simulink model "differentiator"  (R2020b)
settings: Solver=VariableStepAuto  StartTime=0.0  StopTime=0.2  MaxStep=1e-5  RelTol=1e-3  AbsTol=1e-3  EnableMultiTasking=on
libraries: fl_lib x9, nesl_utility x3
CloseFcn:
  | try,close(h1_ssc_opamp_differentiator),end
  | clear h1_ssc_opamp_differentiator
  | clear simlog_ssc_opamp_differentiator
Description:
  | Op-Amp Circuit - Differentiator
settings Model: Creator=The MathWorks, Inc.  LastModifiedBy=bolic
settings SolverCC: AutoScaleAbsTol=off
settings DataIOCC: LimitDataPoints=on  SaveFormat=Array  ReturnWorkspaceOutputs=off
settings OptimizationCC: LifeSpan=inf
settings DebuggingCC: SolverPrmCheckMsg=warning  AllowSymbolicDim=off  PregeneratedLibrarySubsystemCodeDiagnostic=none  SFUnexpectedBacktrackingDiag=warning  SFNoUnconditionalDefaultTransitionDiag=warning  SFExecutionAtInitializationDiag=none  ArithmeticOperatorsInVariantConditions=warning
settings HardwareCC: ProdBitPerPointer=32  ProdBitPerSizeT=32  ProdBitPerPtrDiffT=32  ProdLargestAtomicFloat=None  ProdIntDivRoundTo=Undefined  ProdEndianess=Unspecified  ProdWordSize=32  ProdHWDeviceType=32-bit Generic
settings ModelReferenceCC: PropagateSignalLabelsOutOfModel=off
settings SFSimCC: SimUseLocalCustomCode=off  CustomCodeUndefinedFunction=UseInterfaceOnly
settings RTWCC: RTWUseLocalCustomCode=off
settings CodeAppCC: StateflowObjectComments=on
settings GRTTargetCC: TargetLangStandard=C89/C90 (ANSI)
settings ConfigComp: CovMetricSettings=dw  CovSaveCumulativeToWorkspaceVar=on  CovSaveSingleToWorkspaceVar=on  CovExternalEMLEnable=off  CovSFcnEnable=off
settings SimscapeCC: SimscapeLogType=all  SimscapeLogSimulationStatistics=on  SimscapeLogName=simlog_ssc_opamp_differentiator  SimscapeLogDataHistory=10000

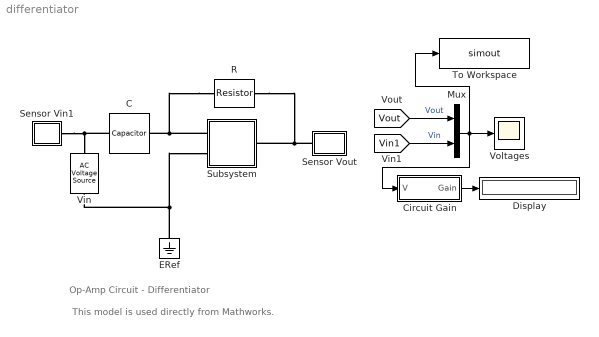
== system differentiator ==
  note: This model is used directly from Mathworks.
  note: Op-Amp Circuit - Differentiator
  C : fl_lib/Electrical/Electrical Elements/Capacitor  c=16 nF  r=1e-6 Ohm  g=0 1/Ohm  i_specify=off  i_priority=High  i=0 A  i_nominal_specify=off  i_nominal_unit=A  i_nominal_value=1  v_specify=off  v_priority=High  v=0 V  v_nominal_specify=off  v_nominal_unit=V  v_nominal_value=1  vc_specify=on  vc_priority=High  vc=0 V  vc_nominal_specify=off  vc_nominal_unit=V  vc_nominal_value=1
      settings: AttributesFormatString=%<C> %<C_unit>  SourceProductName=Foundation Library
  Circuit Gain : Subsystem
  Display : Display
  ERef : fl_lib/Electrical/Electrical Elements/Electrical Reference
      settings: SourceProductName=Foundation Library
  Mux : Mux  Inputs=2
  R : fl_lib/Electrical/Electrical Elements/Resistor  R=100 kOhm  i_specify=off  i_priority=High  i=0 A  i_nominal_specify=off  i_nominal_unit=A  i_nominal_value=1  v_specify=off  v_priority=High  v=0 V  v_nominal_specify=off  v_nominal_unit=V  v_nominal_value=1
      settings: AttributesFormatString=%<R> %<R_unit>  SourceProductName=Foundation Library
  Sensor Vin1 : Subsystem
      mask Display: disp('Vin')
  Sensor Vout : Subsystem
      mask Display: disp('Vo')
  Subsystem : Subsystem
      mask Display: image('op_amp.png')
  To Workspace : ToWorkspace  VariableName=simout  SaveFormat=Timeseries  SampleTime=-1
  Vin : fl_lib/Electrical/Electrical Sources/AC Voltage Source  amp=1 V  shift=0 deg  frequency=10 Hz  omega=0 rad/s
      settings: SourceProductName=Foundation Library
  Voltages : Scope
  wires:
  Mux/1 -> To Workspace/1, Circuit Gain/1(V), Voltages/1
  [Vout] -> Mux/1  "Vout"
  [Vin1] -> Mux/2  "Vin"
  Circuit Gain/1(Gain) -> Display/1
  connections:
  ERef/LConn1 -- Subsystem/LConn2 -- Vin/RConn1
  R/LConn1 -- Subsystem/LConn1 -- C/RConn1
  R/RConn1 -- Sensor Vout/LConn1 -- Subsystem/RConn1
  C/LConn1 -- Sensor Vin1/LConn1 -- Vin/LConn1

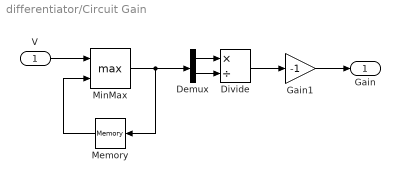
== system differentiator/Circuit Gain ==
  V : Inport
  Demux : Demux  Outputs=2
  Divide : Product  Inputs=*/
  Gain1 : Gain  Gain=-1
  Memory : Memory  InitialCondition=1e-15  InheritSampleTime=on
  MinMax : MinMax  DisableCoverage=on  Function=max  Inputs=2  OutDataTypeStr=Inherit: Inherit via back propagation  ZeroCross=off
      settings: LockScale=on
  Gain : Outport  VectorParamsAs1DForOutWhenUnconnected=off
  wires:
  Gain1/1 -> Gain/1
  Divide/1 -> Gain1/1
  Demux/2 -> Divide/2
  Memory/1 -> MinMax/2
  MinMax/1 -> Demux/1, Memory/1
  Demux/1 -> Divide/1
  V/1 -> MinMax/1

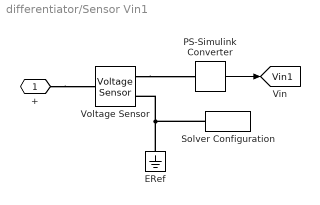
== system differentiator/Sensor Vin1 ==
  ERef : fl_lib/Electrical/Electrical Elements/Electrical Reference
      settings: SourceProductName=Foundation Library
  PS-Simulink Converter : nesl_utility/PS-Simulink Converter  PhysicalDomain=network_engine_domain  SubClassName=ps_output  LeftPortType=input  RightPortType=output  PseudoPeriodic=off  Frequencies=[]  Unit=1  AffineConversion=off
      settings: SourceProductName=Utilities
  Solver Configuration : nesl_utility/Solver Configuration  PhysicalDomain=network_engine_domain  SubClassName=solver  LeftPortType=input  RightPortType=generic  Tones=[]  Harmonics=[]  SimulateNoise=off  Profile=off  UseLocalSampling=off  EnableSwitchedLinearOptims=on  FrequencyDomain=off  UseCCode=off  RelTol=0.001  AbsTol=1e-06  MinStep=1e-09  ToWorkspace=off  RevertToSquareIcSolve=off  NumHomotopyIterations=100  PhasorMode=off  PhasorModeNumHarmonics=1  DoDC=off  ResidualTolerance=1e-9  UseLocalSolver=off  LocalSolverChoice=NE_BACKWARD_EULER_ADVANCER  LocalSolverSampleTime=1e-6  DoFixedCost=off  MaxNonlinIter=3  MaxModeIter=2  ComputeImpulses=off  ImpulseIterations=2  LinearAlgebra=auto  EquationFormulation=NE_TIME_EF  DelaysMemoryBudget=1024  AutomaticFiltering=on  FilteringTimeConstant=0.001  PartitionStorageMethod=AS_NEEDED  PartitionMemoryBudget=1024  PartitionMethod=FAST
      settings: SourceProductName=Utilities
  Voltage Sensor : fl_lib/Electrical/Electrical Sensors/Voltage Sensor
      settings: SourceProductName=Foundation Library
  + : PMIOPort  Side=Left
  tag scope: Vin1=global
  wires:
  PS-Simulink Converter/1 -> [Vin1]
  connections:
  +/RConn1 -- Voltage Sensor/LConn1
  Voltage Sensor/RConn1 -- PS-Simulink Converter/LConn1
  ERef/LConn1 -- Solver Configuration/RConn1 -- Voltage Sensor/RConn2

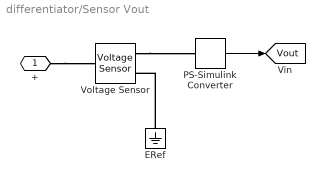
== system differentiator/Sensor Vout ==
  ERef : fl_lib/Electrical/Electrical Elements/Electrical Reference
      settings: SourceProductName=Foundation Library
  PS-Simulink Converter : nesl_utility/PS-Simulink Converter  PhysicalDomain=network_engine_domain  SubClassName=ps_output  LeftPortType=input  RightPortType=output  PseudoPeriodic=off  Frequencies=[]  Unit=1  AffineConversion=off
      settings: SourceProductName=Utilities
  Voltage Sensor : fl_lib/Electrical/Electrical Sensors/Voltage Sensor
      settings: SourceProductName=Foundation Library
  + : PMIOPort  Side=Left
  tag scope: Vout=global
  wires:
  PS-Simulink Converter/1 -> [Vout]
  connections:
  ERef/LConn1 -- Voltage Sensor/RConn2
  Voltage Sensor/RConn1 -- PS-Simulink Converter/LConn1
  +/RConn1 -- Voltage Sensor/LConn1

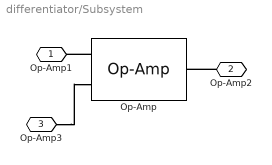
== system differentiator/Subsystem ==
  Op-Amp : fl_lib/Electrical/Electrical Elements/Op-Amp  outI_specify=off  outI_priority=High  outI=0 A  outI_nominal_specify=off  outI_nominal_unit=A  outI_nominal_value=1
      settings: SourceProductName=Foundation Library
  Op-Amp1 : PMIOPort  Side=Left
  Op-Amp2 : PMIOPort  Port=2  Side=Right
  Op-Amp3 : PMIOPort  Port=3  Side=Left
  connections:
  Op-Amp3/RConn1 -- Op-Amp/LConn1
  Op-Amp2/RConn1 -- Op-Amp/RConn1
  Op-Amp/LConn2 -- Op-Amp1/RConn1
